simulink model "sim_fpll"  (R2013b)
settings: Solver=ode45  StartTime=0.0  StopTime=10.0  RelTol=1e-3
libraries: commanapbnd3 x1, commsynccomp2 x1
settings Model: Creator=Kseniya  LastModifiedBy=Kseniya

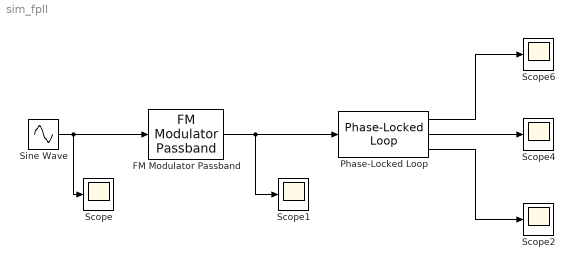
== system sim_fpll ==
  FM Modulator Passband : commanapbnd3/FM Modulator Passband  Fc=200  Ph=0  Kc=20
  Phase-Locked Loop : commsynccomp2/Phase-Locked Loop  Fn="[3.0002  0  40002]"  Fd="[1   67.46   2270.9   40002]"  Kvco=1  Fc=100  Ph=0  Ac=2
  Scope{,1..2,4,6} (5 alike) : Scope
      Scope1 settings: TimeRange=0.2031838875481653  YMin=-2.5  YMax=0
      Scope2 settings: SaveName=ScopeData3
      Scope4 settings: SaveName=ScopeData4
      Scope6 settings: SaveName=ScopeData2
  Sine Wave : Sin  Amplitude=4  Frequency=4  SampleTime=1/300
  wires:
  Sine Wave/1 -> FM Modulator Passband/1, Scope/1
  FM Modulator Passband/1 -> Phase-Locked Loop/1, Scope1/1
  Phase-Locked Loop/2 -> Scope4/1
  Phase-Locked Loop/3 -> Scope2/1
  Phase-Locked Loop/1 -> Scope6/1
